simulink model "regulator_PID_simulink"  (R2025b)
settings: Solver=VariableStepAuto  StartTime=0.0  StopTime=150  RelTol=1e-3
values from neighbouring files (symbols this model uses):
  D_simulink_Bode = Kp_PID_Bode*Td_PID_Bode    [Regulator_PID.m]
  D_simulink_optymalizacja = Kp_optymalizacja*Td_stalaCzasowa    (= 4)    [Regulator_PID.m]
  D_simulink_Tau = Kp_PID_Tau*Td_PID_Tau    [Regulator_PID.m]
  I_simulink_Bode = Kp_PID_Bode/Ti_PID_Bode    [Regulator_PID.m]
  I_simulink_optymalizacja = Kp_optymalizacja/Ti_stalaCzasowa    (= 0.222222222222)    [Regulator_PID.m]
  I_simulink_Tau = Kp_PID_Tau/Ti_PID_Tau    [Regulator_PID.m]
  K_oscylacje = ZapasWzmocnieniaBezwymiarowy_bode    [Regulator_PID.m]
  Kp_optymalizacja = 2    [Regulator_PID.m]
  Kp_PID_Bode = 0.6*K_oscylacje    [Regulator_PID.m]
  Kp_PID_Tau = 1.2*(T/(Kr*tau))    [Regulator_PID.m]
  L1 = [3]    [Regulator_PID.m]
  M1 = conv(m4,m5)    [Regulator_PID.m]
  N = 100    [Regulator_PID.m]
  Sample_time = 0.1    [Regulator_PID.m]
libraries: slpidlib x3
settings Model: LastModifiedBy=mefir

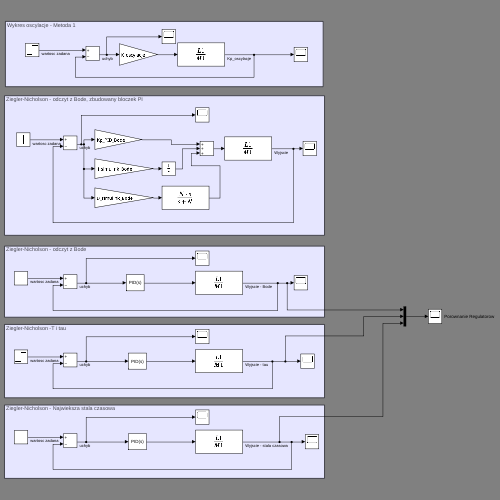
[thumbnail: Simulink's stored preview of the top-level diagram]
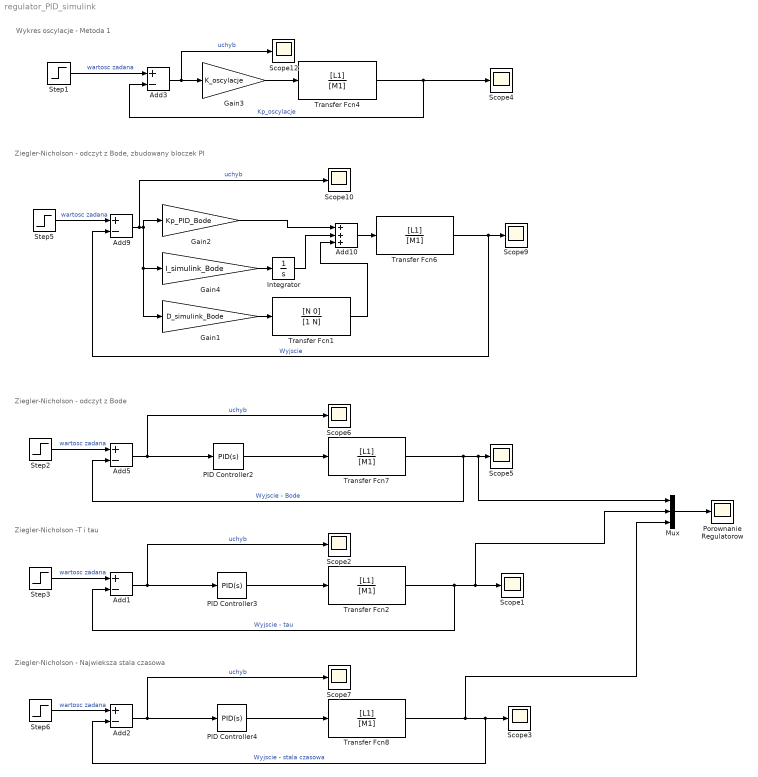
== system regulator_PID_simulink ==
  note: Ziegler-Nicholson - odczyt z Bode, zbudowany bloczek PI
  note: Wykres oscylacje - Metoda 1
  note: Ziegler-Nicholson - odczyt z Bode
  note: Ziegler-Nicholson -T i tau
  note: Ziegler-Nicholson - Najwieksza stala czasowa
  Add{1..3,5,9} (5 alike) : Sum  Inputs=+-
  Add10 : Sum  Inputs=+++
  Gain1 : Gain  Gain=D_simulink_Bode
  Gain2 : Gain  Gain=Kp_PID_Bode
  Gain3 : Gain  Gain=K_oscylacje
  Gain4 : Gain  Gain=I_simulink_Bode
  Integrator : Integrator
  Mux : Mux  Inputs=3
  PID Controller2 : slpidlib/PID Controller  Controller=PID  Form=Parallel  TimeDomain=Continuous-time  UseExternalTs=off  SampleTime=-1  IntegratorMethod=Forward Euler  FilterMethod=Forward Euler  ControllerParametersSource=internal  P=Kp_PID_Bode  I=I_simulink_Bode  UseKiTs=off  D=D_simulink_Bode  UseExternalDerivativeSource=off  N=100  UseFilter=on  TunerSelectOption=Transfer Function Based (PID Tuner App)  InitialConditionSource=internal  InitialConditionForIntegrator=0  InitialConditionForFilter=0  DifferentiatorICPrevScaledInput=0  ExternalReset=none  TrackingMode=off  Kt=1  LimitOutput=off  SatLimitsSource=internal  UpperSaturationLimit=inf  LowerSaturationLimit=-inf  LinearizeAsGain=on  AntiWindupMode=none  Kb=1  LimitIntegrator=off  UpperIntegratorSaturationLimit=inf  LowerIntegratorSaturationLimit=-inf  POutMin=[]  POutMax=[]  IOutMin=[]  IOutMax=[]  DOutMin=[]  DOutMax=[]  NOutMin=[]  NOutMax=[]  SumOutMin=[]  SumOutMax=[]  SaturationOutMin=[]  SaturationOutMax=[]  PParamMin=[]  PParamMax=[]  IParamMin=[]  IParamMax=[]  DParamMin=[]  DParamMax=[]  NParamMin=[]  NParamMax=[]  KbParamMin=[]  KbParamMax=[]  KtParamMin=[]  KtParamMax=[]  KbOutMin=[]  KbOutMax=[]  KtOutMin=[]  KtOutMax=[]  IntegratorOutMin=[]  IntegratorOutMax=[]  FilterOutMin=[]  FilterOutMax=[]  SumI1OutMin=[]  SumI1OutMax=[]  SumI2OutMin=[]  SumI2OutMax=[]  SumI3OutMin=[]  SumI3OutMax=[]  SumI4OutMin=[]  SumI4OutMax=[]  SumDOutMin=[]  SumDOutMax=[]  DifferentiatorOutMin=[]  DifferentiatorOutMax=[]  FilterDiffOutCoefMin=[]  FilterDiffOutCoefMax=[]  ReciprocalOutMin=[]  ReciprocalOutMax=[]  SumDenOutMin=[]  SumDenOutMax=[]  SumNumOutMin=[]  SumNumOutMax=[]  DivideOutMin=[]  DivideOutMax=[]  UdiffTsProdOutMin=[]  UdiffTsProdOutMax=[]  NTsProdOutMin=[]  NTsProdOutMax=[]  UintegralTsProdOutMin=[]  UintegralTsProdOutMax=[]  UngainTsProdOutMin=[]  UngainTsProdOutMax=[]  ClampingZeroOutDataTypeStr=Inherit: Inherit via back propagation  ClampingZeroOutMin=[]  ClampingZeroOutMax=[]  FilterDenConstantOutDataTypeStr=Inherit: Inherit via back propagation  FilterDenConstantOutMin=[]  FilterDenConstantOutMax=[]  PCopyOutDataTypeStr=Inherit: Inherit via back propagation  PCopyOutMin=[]  PCopyOutMax=[]  NCopyOutDataTypeStr=Inherit: Inherit via back propagation  NCopyOutMin=[]  NCopyOutMax=[]  IntegratorContinuousStateAttributes=''  IntegratorStateMustResolveToSignalObject=off  IntegratorRTWStateStorageClass=Auto  FilterContinuousStateAttributes=''  FilterStateMustResolveToSignalObject=off  FilterRTWStateStorageClass=Auto  ParallelPVariant=InternalParameters  IdealPVariant=Disabled  IVariant=InternalParameters  DVariant=InternalParameters  IntegratorVariant=Continuous  SatVariant=Disabled  AWVariant=Passthrough  PCopyVariant=Disabled  TRVariant=Disabled  FdbkBlocksVariant=Forward  IdealPFdbkVariant=Disabled  SatFdbkVariant=Disabled  DerivativeFilterVariant=ContFilter  NVariant=InternalParameters  NCopyVariant=Disabled  FilterICVariant=InternalICsFilter  IntegratorICVariant=InternalICs  ExternalResetVariant=Disabled  TRSumVariant=Passthrough  SumFdbkVariant=Disabled  SumVariant=Sum_PID  TsampFilterVariant=InternalTs  TsampNgainVariant=Passthrough  TsampIntegralVariant=Disabled_SignalSpec  ExternalSaturationOutDataTypeStr=Inherit: Same as second input  DerivativeSourceVariant=ErrorSignal  PreIntVariant=InternalPreInt
  PID Controller3 : slpidlib/PID Controller  Controller=PID  Form=Parallel  TimeDomain=Continuous-time  UseExternalTs=off  SampleTime=-1  IntegratorMethod=Forward Euler  FilterMethod=Forward Euler  ControllerParametersSource=internal  P=Kp_PID_Tau  I=I_simulink_Tau  UseKiTs=off  D=D_simulink_Tau  UseExternalDerivativeSource=off  N=100  UseFilter=on  TunerSelectOption=Transfer Function Based (PID Tuner App)  InitialConditionSource=internal  InitialConditionForIntegrator=0  InitialConditionForFilter=0  DifferentiatorICPrevScaledInput=0  ExternalReset=none  TrackingMode=off  Kt=1  LimitOutput=off  SatLimitsSource=internal  UpperSaturationLimit=inf  LowerSaturationLimit=-inf  LinearizeAsGain=on  AntiWindupMode=none  Kb=1  LimitIntegrator=off  UpperIntegratorSaturationLimit=inf  LowerIntegratorSaturationLimit=-inf  POutMin=[]  POutMax=[]  IOutMin=[]  IOutMax=[]  DOutMin=[]  DOutMax=[]  NOutMin=[]  NOutMax=[]  SumOutMin=[]  SumOutMax=[]  SaturationOutMin=[]  SaturationOutMax=[]  PParamMin=[]  PParamMax=[]  IParamMin=[]  IParamMax=[]  DParamMin=[]  DParamMax=[]  NParamMin=[]  NParamMax=[]  KbParamMin=[]  KbParamMax=[]  KtParamMin=[]  KtParamMax=[]  KbOutMin=[]  KbOutMax=[]  KtOutMin=[]  KtOutMax=[]  IntegratorOutMin=[]  IntegratorOutMax=[]  FilterOutMin=[]  FilterOutMax=[]  SumI1OutMin=[]  SumI1OutMax=[]  SumI2OutMin=[]  SumI2OutMax=[]  SumI3OutMin=[]  SumI3OutMax=[]  SumI4OutMin=[]  SumI4OutMax=[]  SumDOutMin=[]  SumDOutMax=[]  DifferentiatorOutMin=[]  DifferentiatorOutMax=[]  FilterDiffOutCoefMin=[]  FilterDiffOutCoefMax=[]  ReciprocalOutMin=[]  ReciprocalOutMax=[]  SumDenOutMin=[]  SumDenOutMax=[]  SumNumOutMin=[]  SumNumOutMax=[]  DivideOutMin=[]  DivideOutMax=[]  UdiffTsProdOutMin=[]  UdiffTsProdOutMax=[]  NTsProdOutMin=[]  NTsProdOutMax=[]  UintegralTsProdOutMin=[]  UintegralTsProdOutMax=[]  UngainTsProdOutMin=[]  UngainTsProdOutMax=[]  ClampingZeroOutDataTypeStr=Inherit: Inherit via back propagation  ClampingZeroOutMin=[]  ClampingZeroOutMax=[]  FilterDenConstantOutDataTypeStr=Inherit: Inherit via back propagation  FilterDenConstantOutMin=[]  FilterDenConstantOutMax=[]  PCopyOutDataTypeStr=Inherit: Inherit via back propagation  PCopyOutMin=[]  PCopyOutMax=[]  NCopyOutDataTypeStr=Inherit: Inherit via back propagation  NCopyOutMin=[]  NCopyOutMax=[]  IntegratorContinuousStateAttributes=''  IntegratorStateMustResolveToSignalObject=off  IntegratorRTWStateStorageClass=Auto  FilterContinuousStateAttributes=''  FilterStateMustResolveToSignalObject=off  FilterRTWStateStorageClass=Auto  ParallelPVariant=InternalParameters  IdealPVariant=Disabled  IVariant=InternalParameters  DVariant=InternalParameters  IntegratorVariant=Continuous  SatVariant=Disabled  AWVariant=Passthrough  PCopyVariant=Disabled  TRVariant=Disabled  FdbkBlocksVariant=Forward  IdealPFdbkVariant=Disabled  SatFdbkVariant=Disabled  DerivativeFilterVariant=ContFilter  NVariant=InternalParameters  NCopyVariant=Disabled  FilterICVariant=InternalICsFilter  IntegratorICVariant=InternalICs  ExternalResetVariant=Disabled  TRSumVariant=Passthrough  SumFdbkVariant=Disabled  SumVariant=Sum_PID  TsampFilterVariant=InternalTs  TsampNgainVariant=Passthrough  TsampIntegralVariant=Disabled_SignalSpec  ExternalSaturationOutDataTypeStr=Inherit: Same as second input  DerivativeSourceVariant=ErrorSignal  PreIntVariant=InternalPreInt
  PID Controller4 : slpidlib/PID Controller  Controller=PID  Form=Parallel  TimeDomain=Continuous-time  UseExternalTs=off  SampleTime=-1  IntegratorMethod=Forward Euler  FilterMethod=Forward Euler  ControllerParametersSource=internal  P=Kp_optymalizacja  I=I_simulink_optymalizacja  UseKiTs=off  D=D_simulink_optymalizacja  UseExternalDerivativeSource=off  N=100  UseFilter=on  TunerSelectOption=Transfer Function Based (PID Tuner App)  InitialConditionSource=internal  InitialConditionForIntegrator=0  InitialConditionForFilter=0  DifferentiatorICPrevScaledInput=0  ExternalReset=none  TrackingMode=off  Kt=1  LimitOutput=off  SatLimitsSource=internal  UpperSaturationLimit=inf  LowerSaturationLimit=-inf  LinearizeAsGain=on  AntiWindupMode=none  Kb=1  LimitIntegrator=off  UpperIntegratorSaturationLimit=inf  LowerIntegratorSaturationLimit=-inf  POutMin=[]  POutMax=[]  IOutMin=[]  IOutMax=[]  DOutMin=[]  DOutMax=[]  NOutMin=[]  NOutMax=[]  SumOutMin=[]  SumOutMax=[]  SaturationOutMin=[]  SaturationOutMax=[]  PParamMin=[]  PParamMax=[]  IParamMin=[]  IParamMax=[]  DParamMin=[]  DParamMax=[]  NParamMin=[]  NParamMax=[]  KbParamMin=[]  KbParamMax=[]  KtParamMin=[]  KtParamMax=[]  KbOutMin=[]  KbOutMax=[]  KtOutMin=[]  KtOutMax=[]  IntegratorOutMin=[]  IntegratorOutMax=[]  FilterOutMin=[]  FilterOutMax=[]  SumI1OutMin=[]  SumI1OutMax=[]  SumI2OutMin=[]  SumI2OutMax=[]  SumI3OutMin=[]  SumI3OutMax=[]  SumI4OutMin=[]  SumI4OutMax=[]  SumDOutMin=[]  SumDOutMax=[]  DifferentiatorOutMin=[]  DifferentiatorOutMax=[]  FilterDiffOutCoefMin=[]  FilterDiffOutCoefMax=[]  ReciprocalOutMin=[]  ReciprocalOutMax=[]  SumDenOutMin=[]  SumDenOutMax=[]  SumNumOutMin=[]  SumNumOutMax=[]  DivideOutMin=[]  DivideOutMax=[]  UdiffTsProdOutMin=[]  UdiffTsProdOutMax=[]  NTsProdOutMin=[]  NTsProdOutMax=[]  UintegralTsProdOutMin=[]  UintegralTsProdOutMax=[]  UngainTsProdOutMin=[]  UngainTsProdOutMax=[]  ClampingZeroOutDataTypeStr=Inherit: Inherit via back propagation  ClampingZeroOutMin=[]  ClampingZeroOutMax=[]  FilterDenConstantOutDataTypeStr=Inherit: Inherit via back propagation  FilterDenConstantOutMin=[]  FilterDenConstantOutMax=[]  PCopyOutDataTypeStr=Inherit: Inherit via back propagation  PCopyOutMin=[]  PCopyOutMax=[]  NCopyOutDataTypeStr=Inherit: Inherit via back propagation  NCopyOutMin=[]  NCopyOutMax=[]  IntegratorContinuousStateAttributes=''  IntegratorStateMustResolveToSignalObject=off  IntegratorRTWStateStorageClass=Auto  FilterContinuousStateAttributes=''  FilterStateMustResolveToSignalObject=off  FilterRTWStateStorageClass=Auto  ParallelPVariant=InternalParameters  IdealPVariant=Disabled  IVariant=InternalParameters  DVariant=InternalParameters  IntegratorVariant=Continuous  SatVariant=Disabled  AWVariant=Passthrough  PCopyVariant=Disabled  TRVariant=Disabled  FdbkBlocksVariant=Forward  IdealPFdbkVariant=Disabled  SatFdbkVariant=Disabled  DerivativeFilterVariant=ContFilter  NVariant=InternalParameters  NCopyVariant=Disabled  FilterICVariant=InternalICsFilter  IntegratorICVariant=InternalICs  ExternalResetVariant=Disabled  TRSumVariant=Passthrough  SumFdbkVariant=Disabled  SumVariant=Sum_PID  TsampFilterVariant=InternalTs  TsampNgainVariant=Passthrough  TsampIntegralVariant=Disabled_SignalSpec  ExternalSaturationOutDataTypeStr=Inherit: Same as second input  DerivativeSourceVariant=ErrorSignal  PreIntVariant=InternalPreInt
  Porownanie Regulatorow : Scope
      settings: ActiveDisplayYMinimum=-0.59267779679350752  ActiveDisplayYMaximum=2.308362075626202  DataLoggingVariableName=ScopeData7
  Scope{1..7,9..10,12} (10 alike) : Scope
      Scope1 settings: ActiveDisplayYMinimum=-1.1491294790076525  ActiveDisplayYMaximum=2.6607619283357895
      Scope10 settings: ActiveDisplayYMinimum=-1.1491294790076525  ActiveDisplayYMaximum=2.6607619283357895  DataLoggingVariableName=ScopeData10
      Scope12 settings: ActiveDisplayYMinimum=-1.1491294790076525  ActiveDisplayYMaximum=2.6607619283357895  DataLoggingVariableName=ScopeData12
      Scope2 settings: ActiveDisplayYMinimum=-1.1491294790076525  ActiveDisplayYMaximum=2.6607619283357895
      Scope3 settings: ActiveDisplayYMinimum=-1.1491294790076525  ActiveDisplayYMaximum=2.6607619283357895  DataLoggingVariableName=ScopeData2
      Scope4 settings: ActiveDisplayYMinimum=-2.131712214036086  ActiveDisplayYMaximum=2.9033635494589429  DataLoggingVariableName=ScopeData4
      Scope5 settings: ActiveDisplayYMinimum=-1.1491294790076525  ActiveDisplayYMaximum=2.6607619283357895  DataLoggingVariableName=ScopeData5
      Scope6 settings: ActiveDisplayYMinimum=-1.1491294790076525  ActiveDisplayYMaximum=2.6607619283357895  DataLoggingVariableName=ScopeData6
      Scope7 settings: ActiveDisplayYMinimum=-1.1491294790076525  ActiveDisplayYMaximum=2.6607619283357895  DataLoggingVariableName=ScopeData3
      Scope9 settings: ActiveDisplayYMinimum=-4.4435903629035058  ActiveDisplayYMaximum=4.725367576283614  DataLoggingVariableName=ScopeData9
  Step{1..3,5..6} (5 alike) : Step  Time=0  SampleTime=Sample_time
  Transfer Fcn1 : TransferFcn  Numerator=[N 0]  Denominator=[1 N]
  Transfer Fcn{2,4,6..8} (5 alike) : TransferFcn  Numerator=[L1]  Denominator=[M1]
  wires:
  Step1/1 -> Add3/1  "wartosc zadana"
  Add3/1 -> Scope12/1, Gain3/1  "uchyb"
  Transfer Fcn4/1 -> Add3/2, Scope4/1  "Kp_oscylacje"
  Gain3/1 -> Transfer Fcn4/1
  Gain2/1 -> Add10/1
  Transfer Fcn6/1 -> Scope9/1, Add9/2  "Wyjscie"
  Step5/1 -> Add9/1  "wartosc zadana"
  Add9/1 -> Scope10/1, Gain2/1, Gain4/1, Gain1/1  "uchyb"
  Transfer Fcn7/1 -> Mux/1, Scope5/1, Add5/2  "Wyjscie - Bode"
  Step2/1 -> Add5/1  "wartosc zadana"
  Add5/1 -> Scope6/1, PID Controller2/1  "uchyb"
  Add1/1 -> PID Controller3/1, Scope2/1  "uchyb"
  Transfer Fcn2/1 -> Add1/2, Mux/2, Scope1/1  "Wyjscie - tau"
  Step3/1 -> Add1/1  "wartosc zadana"
  PID Controller4/1 -> Transfer Fcn8/1
  Add2/1 -> PID Controller4/1, Scope7/1  "uchyb"
  Transfer Fcn8/1 -> Mux/3, Add2/2, Scope3/1  "Wyjscie - stala czasowa"
  Step6/1 -> Add2/1  "wartosc zadana"
  Mux/1 -> Porownanie Regulatorow/1
  Transfer Fcn1/1 -> Add10/3
  PID Controller2/1 -> Transfer Fcn7/1
  Gain1/1 -> Transfer Fcn1/1
  Integrator/1 -> Add10/2
  Add10/1 -> Transfer Fcn6/1
  PID Controller3/1 -> Transfer Fcn2/1
  Gain4/1 -> Integrator/1
